simulink model "delta_calculation_proposed"  (R2023b)
settings: Solver=ode1  StartTime=0.0  StopTime=0.5  FixedStep=1e-6  RelTol=1e-3
libraries: spsDiodeLib x12, spsIdealSwitchLib x8, spsSeriesRLCBranchLib x5, spsVoltageMeasurementLib x5, spsCurrentMeasurementLib x4, spsLinearTransformerLib x2, spsDCVoltageSourceLib x1, simulink x1, sps_lib x1
settings Model: Creator=lyapunov  LastModifiedBy=lyapunov
settings OptimizationCC: ReuseModelBlockBuffer=off

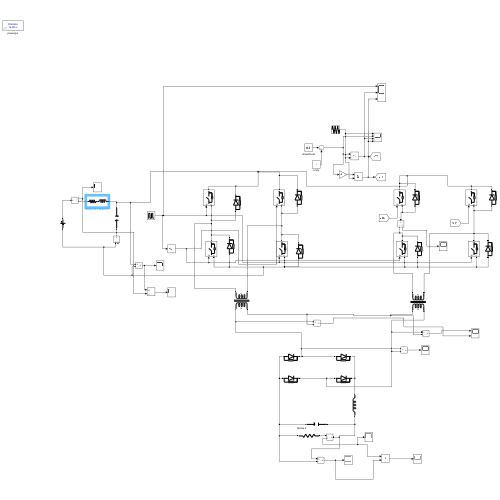
[thumbnail: Simulink's stored preview of the top-level diagram]
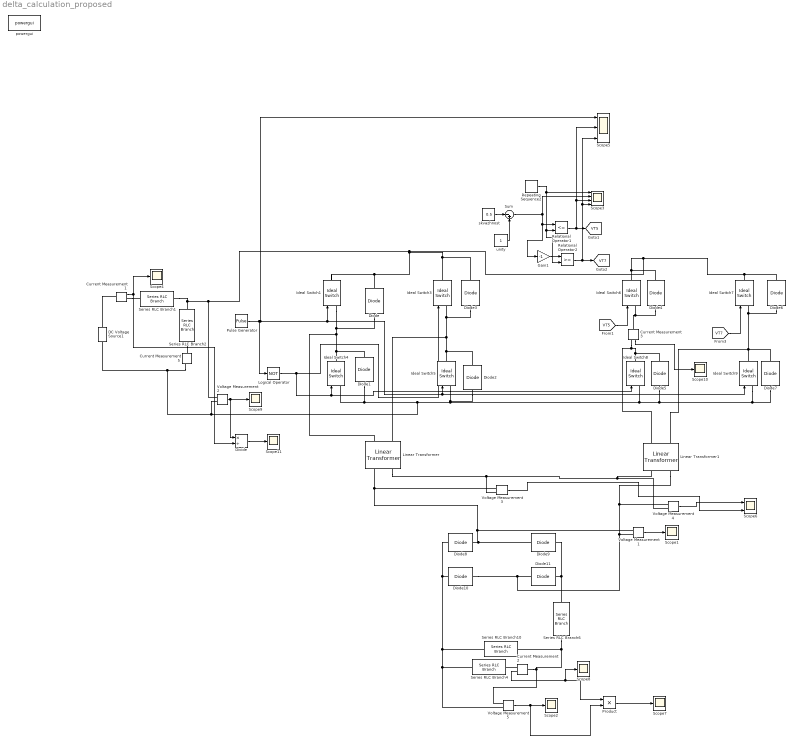
== system delta_calculation_proposed ==
  Current Measurement{1..3,5} (4 alike) : spsCurrentMeasurementLib/Current Measurement  PhasorSimulation=off  OutputType=Complex  PSBequivalent=0
  DC Voltage Source1 : spsDCVoltageSourceLib/DC Voltage Source  Amplitude=300  Measurements=None
  Diode{,1..11} (12 alike) : spsDiodeLib/Diode  Ron=0.001  Lon=0  Vf=0.8  IC=0  UseSnubber=0  Rs=5000  Cs=250e-9  Measurements=off
  Divide : Product  Inputs=*/
  Gain1 : Gain  Gain=-1
  Ideal Switch{1,3..9} (8 alike) : spsIdealSwitchLib/Ideal Switch  Ron=0.001  Lon=0  IC=0  Rs=1e5  Cs=inf  Measurements=off
  Linear Transformer : spsLinearTransformerLib/Linear Transformer  UNITS=SI  NominalPower=[ 500 10000 ]  winding1=[300 0 0]  winding2=[150 0 0]  ThreeWindings=off  winding3=[3.15e+05 0.7938 0.084225]  RmLm=[1e6 1e6]  Measurements=None  DataType=on
  Linear Transformer1 : spsLinearTransformerLib/Linear Transformer  UNITS=SI  NominalPower=[ 500 10000 ]  winding1=[300 0 0]  winding2=[150 0 0]  ThreeWindings=off  winding3=[3.15e+05 0.7938 0.084225]  RmLm=[1e6 1e6]  Measurements=None  DataType=on
  Logical Operator : Logic  Operator=NOT  AllPortsSameDT=off  OutDataTypeStr=boolean
  Product : Product
  Pulse Generator : DiscretePulseGenerator  PulseType=Time based  Period=1/10000  PulseWidth=50
  Relational Operator1 : RelationalOperator  Operator=<=  OutDataTypeStr=boolean  RndMeth=Simplest  InputSameDT=off
  Relational Operator2 : RelationalOperator  OutDataTypeStr=boolean  RndMeth=Simplest  InputSameDT=off
  Repeating Sequence2 : simulink/Sources/Repeating Sequence  rep_seq_t=[0 0.5/20000 1/20000 1.5/20000 2/20000]  rep_seq_y=[0 1 0 -1 0]
  Scope{1..2,4,7..11} (8 alike) : Scope
  Scope3 : Scope  NumInputPorts=4
  Scope5 : Scope  NumInputPorts=3
  Scope6 : Scope  NumInputPorts=2
  Series RLC Branch1 : spsSeriesRLCBranchLib/Series RLC Branch  LConnTagsString=__new0  RConnTagsString=__new0  BranchType=RL  Resistance=0.01  Inductance=11e-04  SetiL0=off  InitialCurrent=0  Capacitance=1e-6  Setx0=off  InitialVoltage=0  Measurements=None
  Series RLC Branch10 : spsSeriesRLCBranchLib/Series RLC Branch  LConnTagsString=__new0  RConnTagsString=__new0  BranchType=C  Resistance=1  Inductance=10e-3  SetiL0=off  InitialCurrent=0  Capacitance=49e-6  Setx0=off  InitialVoltage=0  Measurements=None
  Series RLC Branch2 : spsSeriesRLCBranchLib/Series RLC Branch  LConnTagsString=__new0  RConnTagsString=__new0  BranchType=C  Resistance=1  Inductance=10e-3  SetiL0=off  InitialCurrent=0  Capacitance=6.15e-05  Setx0=off  InitialVoltage=0  Measurements=None
  Series RLC Branch4 : spsSeriesRLCBranchLib/Series RLC Branch  LConnTagsString=__new0  RConnTagsString=__new0  BranchType=R  Resistance=87.23  Inductance=10e-3  SetiL0=off  InitialCurrent=0  Capacitance=100e-6  Setx0=off  InitialVoltage=0  Measurements=None
  Series RLC Branch6 : spsSeriesRLCBranchLib/Series RLC Branch  LConnTagsString=__new0  RConnTagsString=__new0  BranchType=L  Resistance=0.01  Inductance=8e-4  SetiL0=off  InitialCurrent=0  Capacitance=1e-6  Setx0=off  InitialVoltage=0  Measurements=None
  Sum : Sum  Inputs=|-+
  Voltage Measurement{1..5} (5 alike) : spsVoltageMeasurementLib/Voltage Measurement  PhasorSimulation=off  OutputType=Complex  PSBequivalent=0
  powergui : sps_lib/powergui  Priority=1  SimulationMode=Discrete  SampleTime=1e-6  frequency=60  Iterations=50  frequencyindice=0  Pbase=100e6  ErrMax=1e-4  UnitsV=kV  UnitsW=MW  buscounter=0  FunctionMessages=off  echomessages=off  EnableUseOfTLC=off  CurrentSourceSwitches=off  DisableSnubberDevices=off  DisableRonSwitches=off  DisableVfSwitches=off  DisplayEquations=off  AutomaticDiscreteSolvers=off  SolverType=Tustin/Backward Euler (TBE)  Interpol=off  ExternalGateDelay=off  methode=off  Ts=100  x0status=zero  SPID=on  SwTol=0  HookPort=off  NonlinearTolerance=1e-4  nMaxIteration=100  ContinueOnMaxIteration=off  RestoreLinks=warning  ResistiveCurrentMeasurement=off  Frange=[0:2:500]  Ylog=off  Xlog=on  ShowGrid=off  save=off  variable=ZData  structure=0  ZoomFFT=off  StartTime=0.0  cycles=1  DisplayStyle=1  fundamental=60  FreqAxis=off  MaxFrequency=1000  frequencyindicesteady=1  RmsSteady=1  display=off
  skvazhnost : Constant  Value=0.5
  unity : Constant
  tag scope: VT5=global, VT7=global
  wires:
  Pulse Generator/1 -> Logical Operator/1, Scope5/1, Ideal Switch9/1, Ideal Switch5/1, Ideal Switch1/1
  Logical Operator/1 -> Ideal Switch3/1, Ideal Switch8/1, Ideal Switch4/1
  Repeating Sequence2/1 -> Relational Operator2/2, Relational Operator1/2, Scope3/1
  Relational Operator1/1 -> [VT5], Scope5/2, Scope3/3
  Sum/1 -> Gain1/1, Relational Operator1/1, Scope3/2
  Relational Operator2/1 -> Scope5/3, Scope3/4, [VT7]
  Gain1/1 -> Relational Operator2/1
  [VT5] -> Ideal Switch6/1
  [VT7] -> Ideal Switch7/1
  Voltage Measurement4/1 -> Scope6/1
  Voltage Measurement3/1 -> Scope6/2
  Voltage Measurement5/1 -> Product/2, Scope2/1
  skvazhnost/1 -> Sum/1
  unity/1 -> Sum/2
  Voltage Measurement1/1 -> Scope1/1
  Current Measurement1/1 -> Scope4/1, Divide/2
  Current Measurement2/1 -> Scope8/1, Product/1
  Product/1 -> Scope7/1
  Voltage Measurement2/1 -> Divide/1, Scope9/1
  Current Measurement3/1 -> Scope10/1
  Divide/1 -> Scope11/1
  connections:
  Current Measurement1/RConn1 -- Series RLC Branch1/LConn1
  Series RLC Branch2/RConn1 -- Current Measurement5/LConn1
  Current Measurement1/LConn1 -- DC Voltage Source1/RConn1
  Ideal Switch5/RConn1 -- Diode2/RConn1 -- Linear Transformer/LConn1 -- Diode3/LConn1 -- Ideal Switch3/LConn1
  Diode4/LConn1 -- Current Measurement3/LConn1 -- Ideal Switch6/LConn1
  Ideal Switch5/LConn1 -- Diode2/LConn1 -- Diode1/LConn1 -- Ideal Switch4/LConn1 -- DC Voltage Source1/LConn1 -- Current Measurement5/RConn1 -- Voltage Measurement2/LConn2 -- Diode5/LConn1 -- Diode7/LConn1 -- Ideal Switch9/LConn1 -- Ideal Switch8/LConn1
  Ideal Switch1/LConn1 -- Diode/LConn1 -- Linear Transformer/LConn2 -- Diode1/RConn1 -- Ideal Switch4/RConn1
  Ideal Switch9/RConn1 -- Diode7/RConn1 -- Linear Transformer1/LConn1 -- Diode6/LConn1 -- Ideal Switch7/LConn1
  Voltage Measurement4/LConn2 -- Linear Transformer/RConn1 -- Voltage Measurement3/LConn2 -- Linear Transformer1/RConn2
  Voltage Measurement3/LConn1 -- Voltage Measurement1/LConn1 -- Diode8/RConn1 -- Diode9/LConn1 -- Linear Transformer/RConn2
  Linear Transformer1/RConn1 -- Voltage Measurement1/LConn2 -- Diode10/RConn1 -- Diode11/LConn1 -- Voltage Measurement4/LConn1
  Series RLC Branch4/RConn1 -- Voltage Measurement5/LConn2 -- Series RLC Branch10/RConn1 -- Diode8/LConn1 -- Diode10/LConn1
  Current Measurement2/LConn1 -- Voltage Measurement5/LConn1 -- Series RLC Branch10/LConn1 -- Series RLC Branch6/RConn1
  Ideal Switch6/RConn1 -- Diode4/RConn1 -- Voltage Measurement2/LConn1 -- Series RLC Branch1/RConn1 -- Series RLC Branch2/LConn1 -- Diode/RConn1 -- Ideal Switch1/RConn1 -- Diode3/RConn1 -- Ideal Switch3/RConn1 -- Diode6/RConn1 -- Ideal Switch7/RConn1
  Current Measurement2/RConn1 -- Series RLC Branch4/LConn1
  Diode5/RConn1 -- Current Measurement3/RConn1 -- Linear Transformer1/LConn2 -- Ideal Switch8/RConn1
  Diode9/RConn1 -- Series RLC Branch6/LConn1 -- Diode11/RConn1
